simulink model "spring_mass_damp_tf"  (R2021a)
settings: Solver=VariableStepAuto  StartTime=0.0  StopTime=1000  RelTol=1e-3
values from neighbouring files (symbols this model uses):
  B = [0 1/m]'    [spring_mass_func.m]    (also in spring_og_sys.m = [0; 1/m])
  m = 10    [generate_data.m]    (also in spring_og_sys.m; spring_og_sys_id.m; spring_sys_id.m = 5; spring_tf.mat)
undefined symbols (not defined in the file or in its folder): K
libraries: simulink x1
settings Model: Creator=probinet  LastModifiedBy=probinet

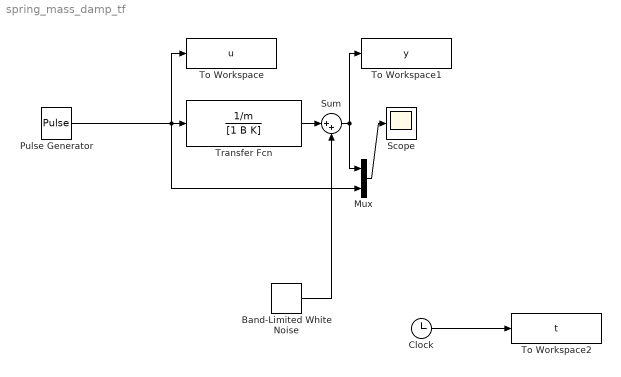
== system spring_mass_damp_tf ==
  Band-Limited White Noise : simulink/Sources/Band-Limited White Noise  Cov=n  Ts=0.1  seed=[23341]
  Clock : Clock
  Mux : Mux  Inputs=2
  Pulse Generator : DiscretePulseGenerator  PulseType=Time based  Period=500  PulseWidth=50
  Scope : Scope
  Sum : Sum  Inputs=|++
  To Workspace : ToWorkspace  VariableName=u  SampleTime=-1
      settings: Save2DSignal=2-D array (concatenate along first dimension)
  To Workspace1 : ToWorkspace  VariableName=y  SampleTime=-1
      settings: Save2DSignal=2-D array (concatenate along first dimension)
  To Workspace2 : ToWorkspace  VariableName=t  SampleTime=-1
      settings: Save2DSignal=2-D array (concatenate along first dimension)
  Transfer Fcn : TransferFcn  Numerator=1/m  Denominator=[1 B K]
  wires:
  Band-Limited White Noise/1 -> Sum/2
  Transfer Fcn/1 -> Sum/1
  Sum/1 -> Mux/1, To Workspace1/1
  Clock/1 -> To Workspace2/1
  Mux/1 -> Scope/1
  Pulse Generator/1 -> To Workspace/1, Transfer Fcn/1, Mux/2
